simulink library "INT_PTOSwt_VD"  (R2016b)
settings: Solver=VariableStepAuto  StartTime=0.0  StopTime=10.0  RelTol=1e-3
settings Model: Creator=bianxuyin  LastModifiedBy=bianxuyin

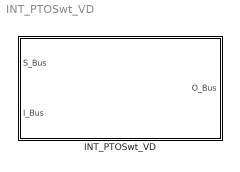
== system INT_PTOSwt_VD ==
  INT_PTOSwt_VD : Subsystem

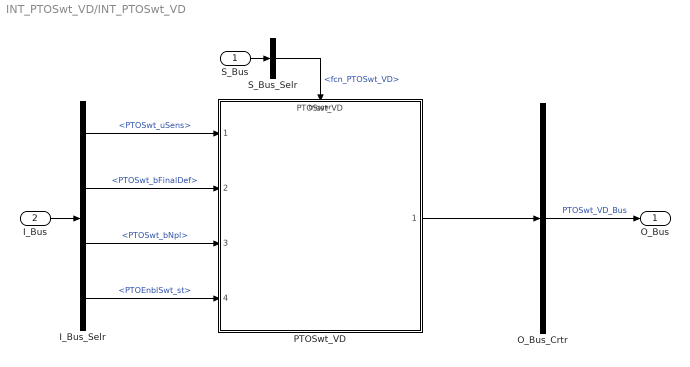
== system INT_PTOSwt_VD/INT_PTOSwt_VD ==
  S_Bus : Inport
  I_Bus : Inport  Port=2
  I_Bus_Selr : BusSelector  OutputSignals=PTOSwt_uSens,PTOSwt_bFinalDef,PTOSwt_bNpl,PTOEnblSwt_st
  O_Bus_Crtr : BusCreator  Inputs=1
  PTOSwt_VD : ModelReference  ModelNameDialog=PTOSwt_VD  SimulationMode=Normal  ModelReferenceVersion=1.15  TriggerPortName=function  TriggerPortTriggerType=function-call  TriggerPortStatesWhenEnabling=held
  S_Bus_Selr : BusSelector  OutputSignals=fcn_PTOSwt_VD
  O_Bus : Outport
  wires:
  S_Bus_Selr/1 -> PTOSwt_VD/Trigger  "<fcn_PTOSwt_VD>"
  S_Bus/1 -> S_Bus_Selr/1
  I_Bus/1 -> I_Bus_Selr/1
  I_Bus_Selr/1 -> PTOSwt_VD/1  "<PTOSwt_uSens>"
  I_Bus_Selr/2 -> PTOSwt_VD/2  "<PTOSwt_bFinalDef>"
  I_Bus_Selr/3 -> PTOSwt_VD/3  "<PTOSwt_bNpl>"
  I_Bus_Selr/4 -> PTOSwt_VD/4  "<PTOEnblSwt_st>"
  O_Bus_Crtr/1 -> O_Bus/1  "PTOSwt_VD_Bus"
  PTOSwt_VD/1 -> O_Bus_Crtr/1
